simulink model "camerainquadrotor_ibvs2016a"  (R2016a)
settings: Solver=ode45  StartTime=0.0  StopTime=10.0  RelTol=1e-3
values from neighbouring files (symbols this model uses):
  ps = cam.project(Marker, 'Tcam', transl(CenterBias'+[0 0 TargetHeight])*trotx(-pi))    [mdl_aerialmanipulator.m]
undefined symbols (not defined in the file or in its folder): aerialmanipulator, pstar, r2t, rpy2tr, transl, trotx
libraries: roblocks x5
settings Model: Creator=zhonghang  LastModifiedBy=dell
settings DataIOCC: LimitDataPoints=on  SaveFormat=Array
settings HardwareCC: ProdBitPerPointer=32  ProdLargestAtomicFloat=None  ProdIntDivRoundTo=Undefined  ProdEndianess=Unspecified  ProdWordSize=32  ProdHWDeviceType=32-bit Generic
settings ModelReferenceCC: PropagateSignalLabelsOutOfModel=off

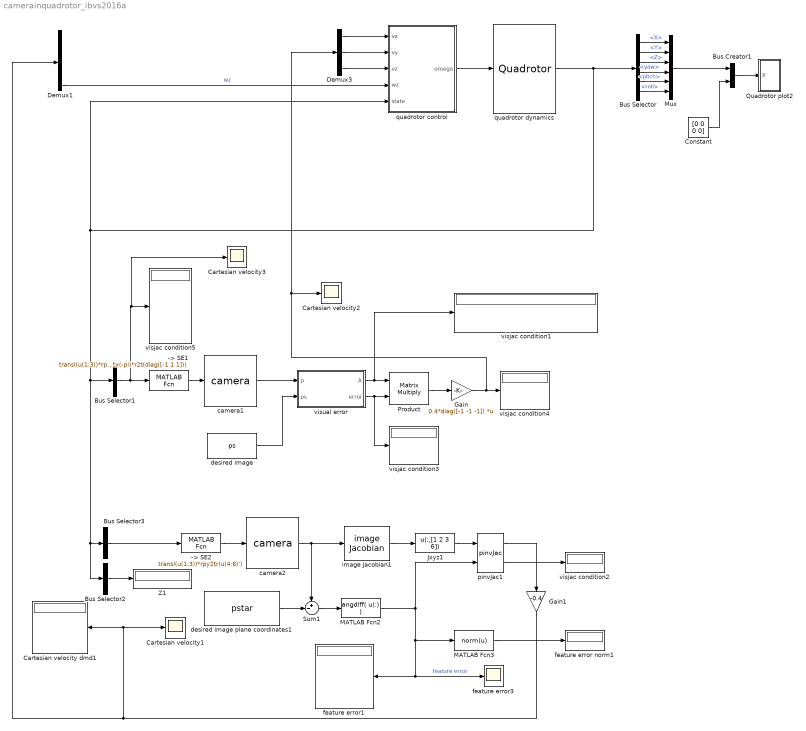
== system camerainquadrotor_ibvs2016a ==
  -> SE1 : MATLABFcn  MATLABFcn=transl(u(1:3))*rpy2tr(u(4:6)')*trotx(-pi)*r2t(diag([-1 1 1]))  OutputDimensions=[4 4]  Output1D=off
  -> SE2 : MATLABFcn  MATLABFcn=transl(u(1:3))*rpy2tr(u(4:6)')  OutputDimensions=[4 4]  Output1D=off
  Bus Creator1 : BusCreator  Inputs=2
  Bus Selector : BusSelector  OutputSignals=X,Y,Z,yaw,pitch,roll
  Bus Selector1 : BusSelector  OutputSignals=X,Y,Z,roll,pitch,yaw  OutputAsBus=on
  Bus Selector2 : BusSelector  OutputSignals=Z  OutputAsBus=on
  Bus Selector3 : BusSelector  OutputSignals=X,Y,Z,roll,pitch,yaw  OutputAsBus=on
  Cartesian velocity dmd1 : Display
      settings: Format=short_e
  Cartesian velocity1 : Scope
  Cartesian velocity2 : Scope
  Cartesian velocity3 : Scope
  Constant : Constant  Value=[0 0 0 0]
  Demux1 : Demux
  Demux3 : Demux  Outputs=3
  Gain : Gain  Gain=0.4*diag([-1 -1 -1])  Multiplication=Matrix(K*u)
  Gain1 : Gain  Gain=-0.4
  Jxyz1 : MATLABFcn  MATLABFcn=u(:,[1 2 3 6])  Output1D=off
  MATLAB Fcn2 : MATLABFcn  MATLABFcn=angdiff( u(:) )  Output1D=off
  MATLAB Fcn3 : MATLABFcn  MATLABFcn=norm(u)
  Mux : Mux  Inputs=6
  Product : Product  Multiplication=Matrix(*)
  Quadrotor plot2 : Subsystem  AncestorBlock=roblocks/Robot Graphics/Quadrotor plot  mask{quad=aerialmanipulator, xydim=1, zdim=10}
      mask prompts: quad "Model"; xydim "xy-axes dimension"; zdim "z-axis dimension"
      mask help: Animate quadrotor.
      mask Help:
      | This block graphically displays a quadrotor (flying robot).
      | 
      | A new figure is created and A graphical model of a quadrotor is animated
      | to a pose specified by the state vector input to the block.
      | 
      | The state vector is [x y z roll pitch yaw] in world coordinates and the
      | angles are in radians.
      | 
      | Notes:
      | - The dimensions of the vehicle workspace are set by parameters
  Sum1 : Sum  Inputs=+-|  SaturateOnIntegerOverflow=on  InputSameDT=on  OutDataTypeStr=Inherit: Same as first input
  Z1 : Display
  camera1 : roblocks/Vision/camera  cam=cam  points=Marker
  camera2 : roblocks/Vision/camera  cam=camera  points=P
  desired image plane coordinates1 : Constant  Value=pstar  VectorParams1D=off
  desired image : Constant  Value=ps  VectorParams1D=off
  feature error norm1 : Display
  feature error1 : Display
      settings: Format=bank
  feature error3 : Scope
  image Jacobian1 : roblocks/Vision/image Jacobian  cam=camera  z=1
  pinvJac1 : roblocks/Vision/pinvJac
  quadrotor control : Subsystem
  quadrotor dynamics : roblocks/Dynamics/Quadrotor  quad=aerialmanipulator
      link override Dynamics: FunctionName=aerialmanipulator_dynamics
  visjac condition{1..5} (5 alike) : Display
  visual error : MATLAB Function  TreatAsAtomicUnit=on
      settings: PermitHierarchicalResolution=ParametersOnly
  wires:
  quadrotor control/1(omega) -> quadrotor dynamics/1
  Bus Creator1/1 -> Quadrotor plot2/1(X)
  Bus Selector/1 -> Mux/1  "<X>"
  Bus Selector/2 -> Mux/2  "<Y>"
  Bus Selector/3 -> Mux/3  "<Z>"
  Bus Selector/4 -> Mux/4  "<yaw>"
  Bus Selector/5 -> Mux/5  "<pitch>"
  Bus Selector/6 -> Mux/6  "<roll>"
  Mux/1 -> Bus Creator1/1
  -> SE1/1 -> camera1/1
  Constant/1 -> Bus Creator1/2
  camera2/1 -> Sum1/1, image Jacobian1/1
  Sum1/1 -> MATLAB Fcn2/1
  desired image plane coordinates1/1 -> Sum1/2
  MATLAB Fcn2/1 -> MATLAB Fcn3/1, feature error1/1, feature error3/1, pinvJac1/2  "feature error"
  image Jacobian1/1 -> Jxyz1/1
  Jxyz1/1 -> pinvJac1/1
  -> SE2/1 -> camera2/1
  Bus Selector3/1 -> -> SE2/1
  MATLAB Fcn3/1 -> feature error norm1/1
  Gain1/1 -> Demux1/1, Cartesian velocity dmd1/1, Cartesian velocity1/1
  Bus Selector2/1 -> Z1/1
  quadrotor dynamics/1 -> Bus Selector/1, quadrotor control/5(state), Bus Selector1/1, Bus Selector2/1, Bus Selector3/1
  pinvJac1/1 -> Gain1/1
  pinvJac1/2 -> visjac condition2/1
  camera1/1 -> visual error/1(p)
  desired image/1 -> visual error/2(ps)
  visual error/1(A) -> visjac condition1/1, Product/1
  Product/1 -> Gain/1
  Gain/1 -> Cartesian velocity2/1, Demux3/1, visjac condition4/1
  visual error/2(error) -> visjac condition3/1, Product/2
  Bus Selector1/1 -> Cartesian velocity3/1, visjac condition5/1, -> SE1/1
  Demux3/1 -> quadrotor control/1(vx)
  Demux3/2 -> quadrotor control/2(vy)
  Demux3/3 -> quadrotor control/3(vz)
  Demux1/4 -> quadrotor control/4(wz)  "wz"

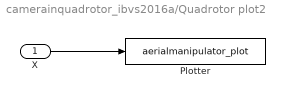
== system camerainquadrotor_ibvs2016a/Quadrotor plot2 ==
  X : Inport
  Plotter : S-Function  FunctionName=aerialmanipulator_plot  Parameters=[xydim, zdim], 1, 1,aerialmanipulator  SFunctionDeploymentMode=off  EnableBusSupport=off
  wires:
  X/1 -> Plotter/1

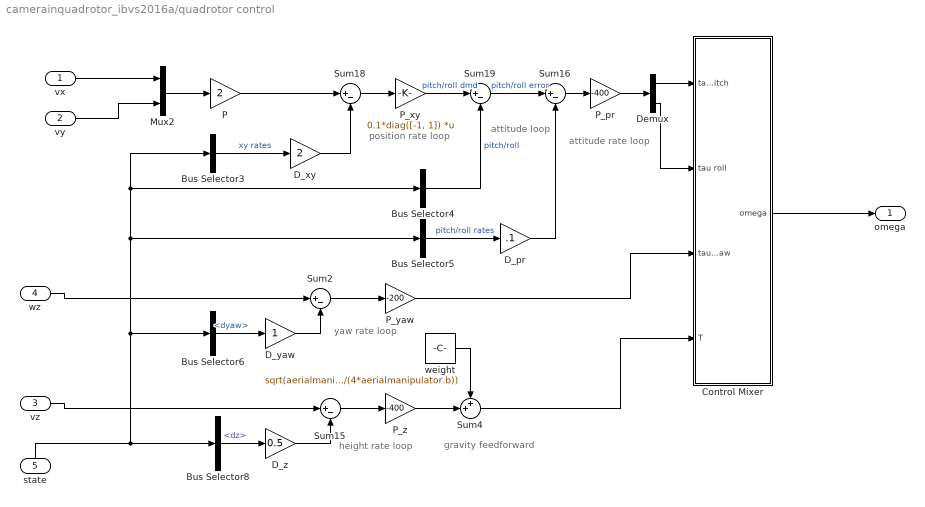
== system camerainquadrotor_ibvs2016a/quadrotor control ==
  note: gravity feedforward
  note: attitude rate
      | loop
  note: attitude
      | loop
  note: position rate
      | loop
  note: yaw rate
      | loop
  note: height rate
      | loop
  vx : Inport
  vy : Inport  Port=2
  vz : Inport  Port=3
  wz : Inport  Port=4
  state : Inport  Port=5
  Bus Selector3 : BusSelector  OutputSignals=dx,dy  OutputAsBus=on
  Bus Selector4 : BusSelector  OutputSignals=pitch,roll  OutputAsBus=on
  Bus Selector5 : BusSelector  OutputSignals=dpitch,droll  OutputAsBus=on
  Bus Selector6 : BusSelector  OutputSignals=dyaw
  Bus Selector8 : BusSelector  OutputSignals=dz
  Control Mixer : Subsystem  AncestorBlock=roblocks/Dynamics/Control Mixer 4
      mask help: Quadrotor control mixer
      mask Help:
      | Determine rotor speeds based on desired torques and thrust.
      | 
      | <b>Inputs::</b>
      | 
      | tau pitch (1x1)  desired pitching torque [Nm]
      | tau roll (1x1)   desired rolling torque [Nm]
      | tau yaw (1x1)    desired yawing torque [Nm]
      | T (1x1)          desired thrust [N]
      | 
      | <b>Outputs::</b>
      | 
      | w1 (1x1) angular velocity of rotor 1 [rad]
      | w2 (1x1) angular velocity of rotor 2 [rad]
      | w3 (1x1) angular velocity of rotor 3 [rad]
      | w4 (1x1) angular velocity of rotor 4 [rad]
      | 
      | <b>Notes::</b>
      | 
      | - Assumes the rotor labelling convention of RVC Fig 4.16.
      | - The quadrotor is underactuated and has only 4 inputs.
  D_pr : Gain  Gain=.1
  D_xy : Gain  Gain=2
  D_yaw : Gain
  D_z : Gain  Gain=0.5
  Demux : Demux  Outputs=2
  Mux2 : Mux  Inputs=2
  P : Gain  Gain=2
  P_pr : Gain  Gain=-400
  P_xy : Gain  Gain=0.1*diag([-1, 1])  Multiplication=Matrix(K*u)
  P_yaw : Gain  Gain=-200
  P_z : Gain  Gain=-400
  Sum{2,15..16,18..19} (5 alike) : Sum  Inputs=|+-
  Sum4 : Sum  Inputs=++|
  weight : Constant  Value=sqrt(aerialmanipulator.M*aerialmanipulator.g/(4*aerialmanipulator.b))  SampleTime=0
  omega : Outport
  wires:
  state/1 -> Bus Selector8/1, Bus Selector5/1, Bus Selector4/1, Bus Selector3/1, Bus Selector6/1
  Mux2/1 -> P/1
  P/1 -> Sum18/1
  Sum18/1 -> P_xy/1
  wz/1 -> Sum2/1
  vz/1 -> Sum15/1
  Control Mixer/1(omega) -> omega/1
  Bus Selector3/1 -> D_xy/1  "xy rates"
  D_xy/1 -> Sum18/2
  P_xy/1 -> Sum19/1  "pitch/roll dmd"
  Bus Selector4/1 -> Sum19/2  "pitch/roll"
  Sum19/1 -> Sum16/1  "pitch/roll error"
  P_pr/1 -> Demux/1
  Bus Selector6/1 -> D_yaw/1  "<dyaw>"
  Bus Selector8/1 -> D_z/1  "<dz>"
  D_z/1 -> Sum15/2
  D_pr/1 -> Sum16/2
  Demux/2 -> Control Mixer/2(tau roll)
  Sum2/1 -> P_yaw/1
  P_yaw/1 -> Control Mixer/3(tau yaw)
  Demux/1 -> Control Mixer/1(tau pitch)
  Bus Selector5/1 -> D_pr/1  "pitch/roll rates"
  D_yaw/1 -> Sum2/2
  weight/1 -> Sum4/1
  Sum4/1 -> Control Mixer/4(T)
  vx/1 -> Mux2/1
  Sum16/1 -> P_pr/1
  vy/1 -> Mux2/2
  Sum15/1 -> P_z/1
  P_z/1 -> Sum4/2

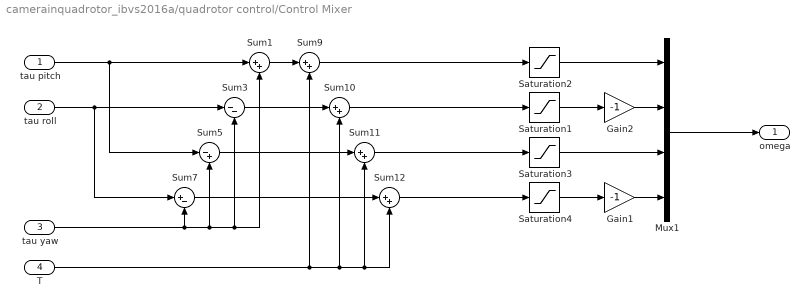
== system camerainquadrotor_ibvs2016a/quadrotor control/Control Mixer ==
  tau pitch : Inport
  tau roll : Inport  Port=2
  tau yaw : Inport  Port=3
  T : Inport  Port=4
  Gain1 : Gain  Gain=-1
  Gain2 : Gain  Gain=-1
  Mux1 : Mux
  Saturation{1..4} (4 alike) : Saturate  UpperLimit=1000  LowerLimit=700
  Sum{1,9..12} (5 alike) : Sum  Inputs=|++  SaturateOnIntegerOverflow=on  InputSameDT=on  OutDataTypeStr=Inherit: Same as first input
  Sum3 : Sum  Inputs=|--  SaturateOnIntegerOverflow=on  InputSameDT=on  OutDataTypeStr=Inherit: Same as first input
  Sum5 : Sum  Inputs=|-+  SaturateOnIntegerOverflow=on  InputSameDT=on  OutDataTypeStr=Inherit: Same as first input
  Sum7 : Sum  Inputs=|+-  SaturateOnIntegerOverflow=on  InputSameDT=on  OutDataTypeStr=Inherit: Same as first input
  omega : Outport
  wires:
  Mux1/1 -> omega/1
  Gain2/1 -> Mux1/2
  tau yaw/1 -> Sum7/2, Sum5/2, Sum3/2, Sum1/2
  Saturation2/1 -> Mux1/1
  Saturation1/1 -> Gain2/1
  Saturation3/1 -> Mux1/3
  Saturation4/1 -> Gain1/1
  tau pitch/1 -> Sum1/1, Sum5/1
  Sum1/1 -> Sum9/1
  Sum3/1 -> Sum10/1
  Sum5/1 -> Sum11/1
  Sum7/1 -> Sum12/1
  Sum9/1 -> Saturation2/1
  Sum10/1 -> Saturation1/1
  Sum11/1 -> Saturation3/1
  Sum12/1 -> Saturation4/1
  T/1 -> Sum11/2, Sum12/2, Sum10/2, Sum9/2
  tau roll/1 -> Sum3/1, Sum7/1
  Gain1/1 -> Mux1/4

== matlab function camerainquadrotor_ibvs2016a/visual error ==
  data: A output; p input; error output; ps input
function [A, error] = visualerror(p, ps)
%% get the visual error message
% cal s and s*
[m,n] = size(p);
s = (1/500)*(p - repmat([640;400],[1 n]));
s = [s; ones(1,n)];
for i=1:n
    s(:,i) = s(:,i)./norm(s(:,i));
end
st = (1/500)*(ps - repmat([640;400],[1 n]));
st = [st; ones(1,n)];
for i=1:n
    st(:,i) = st(:,i)./norm(st(:,i));
end
% cal sum of s
h = sum(s,2);
ht = sum(st,2);
% delta h 
delta_h = h - ht;
%% modefied delta h
namda = 2;
ht_stat = ht./norm(ht);
% error = h - ht;
error = cross(ht_stat, h) + namda*ht_stat*(ht_stat'*delta_h);
%% A for use
sk_ht = [0 -ht_stat(3) ht_stat(2);...
    ht_stat(3) 0 -ht_stat(1);...
    -ht_stat(2) ht_stat(1) 0];
A = -sk_ht + namda*(ht_stat*ht_stat');
